simulink model "lin_model_PI_MRAC_Sim_CASE1"  (Simulink 7.7)
settings: Solver=ode45  StartTime=0.0  StopTime=TIME  RelTol=1e-3  AbsTol=1e-6
values from neighbouring files (symbols this model uses):
  Am = AA - BB*Kr    [lin_model_LQR.m]    (also in lin_model_PI_MRAC_CASE1.m = Ar-BB*Kr; lin_model_PI_MRAC_CASE1_L1.m = Ar-BB*Kr)
  Ar = Ar_cruise    [parameter.m]
  BB = B_cruise    [parameter.m]
  bm = -(CC*inv(Am))\eye(11)    [lin_model_PI_MRAC_CASE1.m]    (also in lin_model_PI_MRAC_CASE1_L1.m)
  gamma = rho*c_cr*a_cr*(r_cr)^4/Icr    (= 0.431761992187)    [beta_crS.m]    (also in heli_parameter.m = 5.40374741035; lin_model_PI_MRAC_CASE1.m = 1000000; lin_model_PI_MRAC_CASE1_L1.m = 10000; parameter.m = 5.40374741035)
  noise = 0.1    [lin_model_PI_MRAC_CASE1_L1.m]
  Theta_a = AA-Ar    [parameter.m]
  theta_hat0 = eye(11)    [lin_model_PI_MRAC_CASE1.m]    (also in lin_model_PI_MRAC_CASE1_L1.m)
  x0 = [0;0;0;0]    [beta_crS.m]    (also in flapping.m = []; flappingthrust.m = []; lin_flapping.m = []; lin_model_LQR.m = [3 3 3 0 0 0 0 0 0 0 0]')
  x_hat0 = x0    [lin_model_PI_MRAC_CASE1.m]    (also in lin_model_PI_MRAC_CASE1_L1.m)
undefined symbols (not defined in the file or in its folder): Kr
libraries: simulink x1, commnoisgen2 x1
settings Model: Creator=Li  LastModifiedBy=Li
settings DataIOCC: LimitDataPoints=off  SaveFormat=Structure
settings DebuggingCC: SolverPrmCheckMsg=none

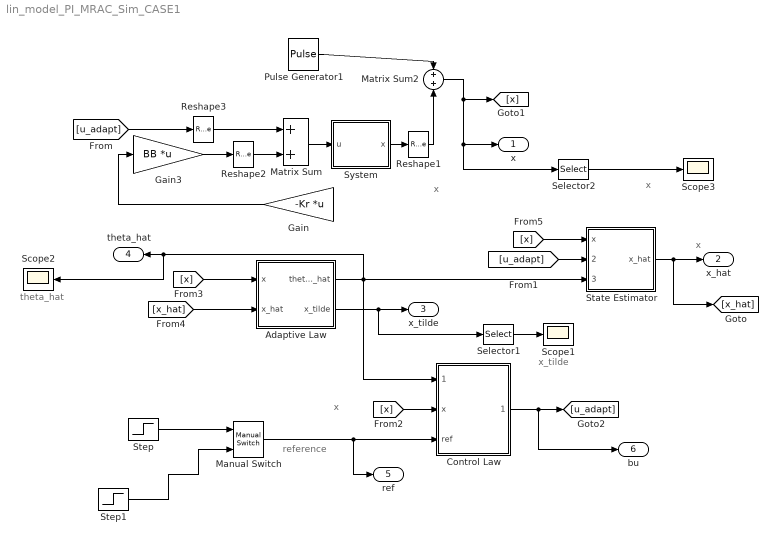
== system lin_model_PI_MRAC_Sim_CASE1 ==
  note: x
  note: x
  note: reference
  note: theta_hat
  note: x_tilde
  note: x
  note: x
  Adaptive Law : Subsystem
  Control Law : Subsystem
  Gain : Gain  Gain=-Kr  Multiplication=Matrix(K*u) (u vector)
  Gain3 : Gain  Gain=BB  Multiplication=Matrix(K*u) (u vector)
  Manual Switch : simulink/Signal Routing/Manual Switch  SystemSampleTime=-1  sw=1  action=0  varsize=off
  Matrix Sum : Sum
  Matrix Sum2 : Sum
  Pulse Generator1 : DiscretePulseGenerator  PulseType=Time based  Amplitude="[0  0 0 0 0 0 0 0 0 0 0];"  Period=7  PhaseDelay=3
  Reshape1 : Reshape  OutputDimensionality=Column vector (2-D)
  Reshape2 : Reshape  OutputDimensionality=Column vector (2-D)
  Reshape3 : Reshape  OutputDimensionality=Column vector (2-D)
  Scope1 : Scope
      settings: TimeRange=3  YMin=-3e+007  YMax=2.5e+006
  Scope2 : Scope
      settings: TimeRange=20  YMin=-1  YMax=1
  Scope3 : Scope
      settings: TimeRange=20  YMin=-7.5  YMax=17.5  SaveName=ScopeData2
  Selector1 : Selector  InputPortWidth=11  IndexOptions=Index vector (dialog)  Indices=[1 2 3 4 5]  OutputSizes=1
  Selector2 : Selector  InputPortWidth=11  IndexOptions=Index vector (dialog)  Indices=[1 2 3]  OutputSizes=1
  State Estimator : Subsystem
  Step : Step  Time=5  Before=[15 0 0 0 0 0 0 0 0 0 0]'  After=[10 -5 2 0 0 0 0 0 0 0 0]'  SampleTime=0
  Step1 : Step  Time=0  After=[0 0 0 0 0 0 0 0 0 0 0]'  SampleTime=0
  System : Subsystem
  x : Outport
  x_hat : Outport  Port=2
  x_tilde : Outport  Port=3
  theta_hat : Outport  Port=4
  ref : Outport  Port=5
  bu : Outport  Port=6
  wires:
  Matrix Sum/1 -> System/1(u)
  State Estimator/1(x_hat) -> x_hat/1, [x_hat]
  [u_adapt] -> State Estimator/2(u_adapt)
  Gain/1 -> Gain3/1
  [x] -> Adaptive Law/1(x)
  [x_hat] -> Adaptive Law/2(x_hat)
  Adaptive Law/1(theta_hat) -> State Estimator/3(theta_hat), Control Law/1(theta_hat), theta_hat/1, Scope2/1
  Control Law/1(u_adap) -> [u_adapt], bu/1
  Step/1 -> Manual Switch/1
  Manual Switch/1 -> Control Law/3(ref), ref/1
  System/1(x) -> Reshape1/1
  Gain3/1 -> Reshape2/1
  Reshape2/1 -> Matrix Sum/2
  [u_adapt] -> Reshape3/1
  Reshape3/1 -> Matrix Sum/1
  Selector1/1 -> Scope1/1
  Adaptive Law/2(x_tilde) -> x_tilde/1, Selector1/1
  Selector2/1 -> Scope3/1
  [x] -> Control Law/2(x)
  [x] -> State Estimator/1(x)
  Step1/1 -> Manual Switch/2
  Pulse Generator1/1 -> Matrix Sum2/1
  Reshape1/1 -> Matrix Sum2/2
  Matrix Sum2/1 -> [x], x/1, Selector2/1

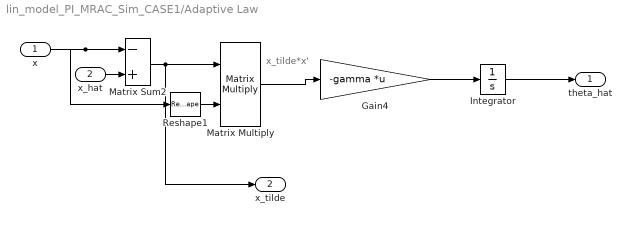
== system lin_model_PI_MRAC_Sim_CASE1/Adaptive Law ==
  note: x_tilde*x'
  x : Inport
  x_hat : Inport  Port=2
  Gain4 : Gain  Gain=-gamma  Multiplication=Matrix(K*u)
  Integrator : Integrator  InitialCondition=theta_hat0
  Matrix Sum2 : Sum  Inputs=-+
  Matrix Multiply : Product  Multiplication=Matrix(*)
  Reshape1 : Reshape  OutputDimensionality=Row vector (2-D)
  theta_hat : Outport
  x_tilde : Outport  Port=2
  wires:
  Matrix Sum2/1 -> Matrix Multiply/1, x_tilde/1
  Reshape1/1 -> Matrix Multiply/2
  Matrix Multiply/1 -> Gain4/1
  x/1 -> Matrix Sum2/1, Reshape1/1
  x_hat/1 -> Matrix Sum2/2
  Gain4/1 -> Integrator/1
  Integrator/1 -> theta_hat/1

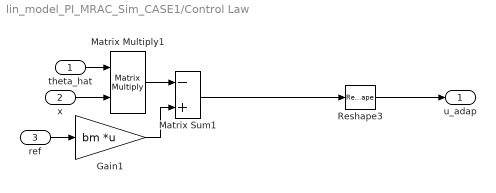
== system lin_model_PI_MRAC_Sim_CASE1/Control Law ==
  theta_hat : Inport
  x : Inport  Port=2
  ref : Inport  Port=3
  Gain1 : Gain  Gain=bm  Multiplication=Matrix(K*u) (u vector)
  Matrix Sum1 : Sum  Inputs=-+
  Matrix Multiply1 : Product  Multiplication=Matrix(*)
  Reshape3 : Reshape  OutputDimensionality=Column vector (2-D)
  u_adap : Outport
  wires:
  Matrix Multiply1/1 -> Matrix Sum1/1
  Gain1/1 -> Matrix Sum1/2
  x/1 -> Matrix Multiply1/2
  theta_hat/1 -> Matrix Multiply1/1
  ref/1 -> Gain1/1
  Reshape3/1 -> u_adap/1
  Matrix Sum1/1 -> Reshape3/1

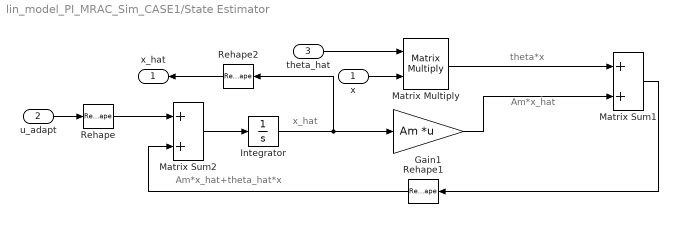
== system lin_model_PI_MRAC_Sim_CASE1/State Estimator ==
  note: x_hat
  note: theta*x
  note: Am*x_hat
  note: Am*x_hat+theta_hat*x
  x : Inport
  u_adapt : Inport  Port=2
  theta_hat : Inport  Port=3
  Gain1 : Gain  Gain=Am  Multiplication=Matrix(K*u) (u vector)
  Integrator : Integrator  InitialCondition=x_hat0
  Matrix Sum1 : Sum
  Matrix Sum2 : Sum
  Matrix Multiply : Product  Multiplication=Matrix(*)
  Rehape : Reshape  OutputDimensionality=Column vector (2-D)
  Rehape1 : Reshape  OutputDimensionality=Column vector (2-D)
  Rehape2 : Reshape  OutputDimensionality=Column vector (2-D)
  x_hat : Outport
  wires:
  theta_hat/1 -> Matrix Multiply/1
  Integrator/1 -> Gain1/1, Rehape2/1
  Matrix Multiply/1 -> Matrix Sum1/1
  Gain1/1 -> Matrix Sum1/2
  Matrix Sum2/1 -> Integrator/1
  x/1 -> Matrix Multiply/2
  Rehape/1 -> Matrix Sum2/1
  u_adapt/1 -> Rehape/1
  Matrix Sum1/1 -> Rehape1/1
  Rehape1/1 -> Matrix Sum2/2
  Rehape2/1 -> x_hat/1

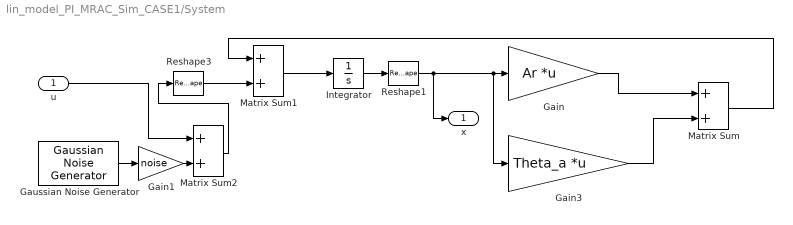
== system lin_model_PI_MRAC_Sim_CASE1/System ==
  u : Inport
  Gain : Gain  Gain=Ar  Multiplication=Matrix(K*u) (u vector)
  Gain1 : Gain  Gain=noise
  Gain3 : Gain  Gain=Theta_a  Multiplication=Matrix(K*u) (u vector)
  Gaussian Noise Generator : commnoisgen2/Gaussian Noise Generator  SystemSampleTime=-1  m=0  d=5*ones(11,1)  s=41  Ts=1  frameBased=off  sampPerFrame=1  orient=off  outDataType=double
  Integrator : Integrator  InitialCondition=x0
  Matrix Sum : Sum
  Matrix Sum1 : Sum
  Matrix Sum2 : Sum
  Reshape1 : Reshape  OutputDimensionality=Column vector (2-D)
  Reshape3 : Reshape  OutputDimensionality=Column vector (2-D)
  x : Outport
  wires:
  Gain/1 -> Matrix Sum/1
  Gain3/1 -> Matrix Sum/2
  Matrix Sum1/1 -> Integrator/1
  Matrix Sum/1 -> Matrix Sum1/1
  Integrator/1 -> Reshape1/1
  Reshape1/1 -> Gain3/1, Gain/1, x/1
  Matrix Sum2/1 -> Reshape3/1
  Reshape3/1 -> Matrix Sum1/2
  u/1 -> Matrix Sum2/1
  Gaussian Noise Generator/1 -> Gain1/1
  Gain1/1 -> Matrix Sum2/2
